simulink model "sim_battery_pack_simulink_18_11"  (R2021a)
settings: Solver=FixedStepAuto  StartTime=0.0  StopTime=3460.480  FixedStep=0.01  RelTol=1e-3
values from neighbouring files (symbols this model uses):
  Af = 1.4*1.6    (= 2.24)    [battery_pack_init_18_11.m]
  b = 0.002    [battery_pack_init_18_11.m]
  Batt_Eff = .98    (= 0.98)    [battery_pack_init_18_11.m]
  Batt_Ene_Cap = 7.37    [battery_pack_init_18_11.m]
  cd = 0.45    [battery_pack_init_18_11.m]
  dt = 0.01    [battery_pack_init_18_11.m]
  g = 9.81    [battery_pack_init_18_11.m]
  Gr = 5.75*.85    (= 4.8875)    [battery_pack_init_18_11.m]
  Grade = 7    [battery_pack_init_18_11.m]
  Ini_SOC = 100    [battery_pack_init_18_11.m]
  kappa = 0.1    [battery_pack_init_18_11.m]
  M = M_k+M_P    (= 445)    [battery_pack_init_18_11.m]
  M_Trq = T_m    [battery_pack_init_18_11.m]
  M_w = w_m    [battery_pack_init_18_11.m]
  Mot_Eff = .9    (= 0.9)    [battery_pack_init_18_11.m]
  mu = 0.016    [battery_pack_init_18_11.m]
  Np = 7    [battery_pack_init_18_11.m]
  Ns = 12    [battery_pack_init_18_11.m]
  Qgain = 1    [battery_pack_init_18_11.m]
  R0 = zeros(numpoles,1)    [battery_pack_init_18_11.m]
  R0Param = getParamESC('R0Param',T,cell_model)    [battery_pack_init_18_11.m]
  R_w = .3048/2    (= 0.1524)    [battery_pack_init_18_11.m]
  Re_spe_max = 50*5/18    (= 13.8888888889)    [battery_pack_init_18_11.m]
  Re_spe_min = 0*5/18    (= 0)    [battery_pack_init_18_11.m]
  rho = 1.225    [battery_pack_init_18_11.m]
  rt = .0008    (= 0.0008)    [battery_pack_init_18_11.m]
  T = 40    [battery_pack_init_18_11.m]
  T_MIDC = T_MIDC(1:72)    [battery_pack_init_18_11.m]
  Trans_Eff = .95    (= 0.95)    [battery_pack_init_18_11.m]
  V_MIDC = V_MIDC(1:72)    [battery_pack_init_18_11.m]
  Z0 = 0.75 + (1-0.75).*rand(1,Np)    [battery_pack_init_18_11.m]
undefined symbols (not defined in the file or in its folder): cell_model, FLbattery, gain, iload, sigbuilder_block, VMIDC
libraries: simulink x16, autolibshared x2, pid_lib x1, simulink_extras x1
(part 2 of 17)

== system sim_battery_pack_simulink_18_11/SCM3/cell2 ==
  ik1 : Inport
  Constant : Constant  Value=R0
  Constant1 : Constant  Value=dt
  Constant2 : Constant  Value=T
  States : Scope  NumInputPorts=2
  Unit Delay : UnitDelay  InitialCondition=Z0(2,3)  SampleTime=-1  HasFrameUpgradeWarning=on
  Unit Delay1 : UnitDelay  SampleTime=-1  HasFrameUpgradeWarning=on
  Voltage : Scope  NumInputPorts=2
  cell_model : MATLAB Function  TreatAsAtomicUnit=on
  V1 : Outport
  Z1 : Outport  Port=2
  irc1 : Outport  Port=3
  wires:
  cell_model/4(OCV) -> Voltage/2
  ik1/1 -> cell_model/6(ik)
  cell_model/3(zkc) -> Z1/1, Unit Delay/1, States/1
  cell_model/1(vk) -> V1/1, Voltage/1
  Constant1/1 -> cell_model/2(deltaT)
  Constant2/1 -> cell_model/1(T)
  Unit Delay/1 -> cell_model/4(zkp)
  cell_model/2(irkc) -> irc1/1, Unit Delay1/1, States/2
  Unit Delay1/1 -> cell_model/5(irkp)
  Constant/1 -> cell_model/3(iR0)

== system sim_battery_pack_simulink_18_11/SCM3/cell3 ==
  ik1 : Inport
  Constant : Constant  Value=R0
  Constant1 : Constant  Value=dt
  Constant2 : Constant  Value=T
  States : Scope  NumInputPorts=2
  Unit Delay : UnitDelay  InitialCondition=Z0(3,3)  SampleTime=-1  HasFrameUpgradeWarning=on
  Unit Delay1 : UnitDelay  SampleTime=-1  HasFrameUpgradeWarning=on
  Voltage : Scope  NumInputPorts=2
  cell_model : MATLAB Function  TreatAsAtomicUnit=on
  V1 : Outport
  Z1 : Outport  Port=2
  irc1 : Outport  Port=3
  wires:
  Constant/1 -> cell_model/3(iR0)
  Unit Delay1/1 -> cell_model/5(irkp)
  cell_model/2(irkc) -> States/2, Unit Delay1/1, irc1/1
  Unit Delay/1 -> cell_model/4(zkp)
  Constant2/1 -> cell_model/1(T)
  Constant1/1 -> cell_model/2(deltaT)
  cell_model/1(vk) -> Voltage/1, V1/1
  cell_model/3(zkc) -> States/1, Unit Delay/1, Z1/1
  ik1/1 -> cell_model/6(ik)
  cell_model/4(OCV) -> Voltage/2

== system sim_battery_pack_simulink_18_11/SCM3/cell4 ==
  ik1 : Inport
  Constant : Constant  Value=R0
  Constant1 : Constant  Value=dt
  Constant2 : Constant  Value=T
  States : Scope  NumInputPorts=2
  Unit Delay : UnitDelay  InitialCondition=Z0(4,3)  SampleTime=-1  HasFrameUpgradeWarning=on
  Unit Delay1 : UnitDelay  SampleTime=-1  HasFrameUpgradeWarning=on
  Voltage : Scope  NumInputPorts=2
  cell_model : MATLAB Function  TreatAsAtomicUnit=on
  V1 : Outport
  Z1 : Outport  Port=2
  irc1 : Outport  Port=3
  wires:
  Constant/1 -> cell_model/3(iR0)
  Unit Delay1/1 -> cell_model/5(irkp)
  cell_model/2(irkc) -> States/2, Unit Delay1/1, irc1/1
  Unit Delay/1 -> cell_model/4(zkp)
  Constant2/1 -> cell_model/1(T)
  Constant1/1 -> cell_model/2(deltaT)
  cell_model/1(vk) -> Voltage/1, V1/1
  cell_model/3(zkc) -> States/1, Unit Delay/1, Z1/1
  ik1/1 -> cell_model/6(ik)
  cell_model/4(OCV) -> Voltage/2

== system sim_battery_pack_simulink_18_11/SCM3/cell5 ==
  ik1 : Inport
  Constant : Constant  Value=R0
  Constant1 : Constant  Value=dt
  Constant2 : Constant  Value=T
  States : Scope  NumInputPorts=2
  Unit Delay : UnitDelay  InitialCondition=Z0(5,3)  SampleTime=-1  HasFrameUpgradeWarning=on
  Unit Delay1 : UnitDelay  SampleTime=-1  HasFrameUpgradeWarning=on
  Voltage : Scope  NumInputPorts=2
  cell_model : MATLAB Function  TreatAsAtomicUnit=on
  V1 : Outport
  Z1 : Outport  Port=2
  irc1 : Outport  Port=3
  wires:
  cell_model/4(OCV) -> Voltage/2
  ik1/1 -> cell_model/6(ik)
  cell_model/3(zkc) -> Z1/1, Unit Delay/1, States/1
  cell_model/1(vk) -> V1/1, Voltage/1
  Constant1/1 -> cell_model/2(deltaT)
  Constant2/1 -> cell_model/1(T)
  Unit Delay/1 -> cell_model/4(zkp)
  cell_model/2(irkc) -> irc1/1, Unit Delay1/1, States/2
  Unit Delay1/1 -> cell_model/5(irkp)
  Constant/1 -> cell_model/3(iR0)

== system sim_battery_pack_simulink_18_11/SCM3/cell6 ==
  ik1 : Inport
  Constant : Constant  Value=R0
  Constant1 : Constant  Value=dt
  Constant2 : Constant  Value=T
  States : Scope  NumInputPorts=2
  Unit Delay : UnitDelay  InitialCondition=Z0(6,3)  SampleTime=-1  HasFrameUpgradeWarning=on
  Unit Delay1 : UnitDelay  SampleTime=-1  HasFrameUpgradeWarning=on
  Voltage : Scope  NumInputPorts=2
  cell_model : MATLAB Function  TreatAsAtomicUnit=on
  V1 : Outport
  Z1 : Outport  Port=2
  irc1 : Outport  Port=3
  wires:
  cell_model/4(OCV) -> Voltage/2
  ik1/1 -> cell_model/6(ik)
  cell_model/3(zkc) -> Z1/1, Unit Delay/1, States/1
  cell_model/1(vk) -> V1/1, Voltage/1
  Constant1/1 -> cell_model/2(deltaT)
  Constant2/1 -> cell_model/1(T)
  Unit Delay/1 -> cell_model/4(zkp)
  cell_model/2(irkc) -> irc1/1, Unit Delay1/1, States/2
  Unit Delay1/1 -> cell_model/5(irkp)
  Constant/1 -> cell_model/3(iR0)

== system sim_battery_pack_simulink_18_11/SCM3/cell7 ==
  ik1 : Inport
  Constant : Constant  Value=R0
  Constant1 : Constant  Value=dt
  Constant2 : Constant  Value=T
  States : Scope  NumInputPorts=2
  Unit Delay : UnitDelay  InitialCondition=Z0(7,3)  SampleTime=-1  HasFrameUpgradeWarning=on
  Unit Delay1 : UnitDelay  SampleTime=-1  HasFrameUpgradeWarning=on
  Voltage : Scope  NumInputPorts=2
  cell_model : MATLAB Function  TreatAsAtomicUnit=on
  V1 : Outport
  Z1 : Outport  Port=2
  irc1 : Outport  Port=3
  wires:
  Constant/1 -> cell_model/3(iR0)
  Unit Delay1/1 -> cell_model/5(irkp)
  cell_model/2(irkc) -> States/2, Unit Delay1/1, irc1/1
  Unit Delay/1 -> cell_model/4(zkp)
  Constant2/1 -> cell_model/1(T)
  Constant1/1 -> cell_model/2(deltaT)
  cell_model/1(vk) -> Voltage/1, V1/1
  cell_model/3(zkc) -> States/1, Unit Delay/1, Z1/1
  ik1/1 -> cell_model/6(ik)
  cell_model/4(OCV) -> Voltage/2

== system sim_battery_pack_simulink_18_11/SCM3/cell8 ==
  ik1 : Inport
  Constant : Constant  Value=R0
  Constant1 : Constant  Value=dt
  Constant2 : Constant  Value=T
  States : Scope  NumInputPorts=2
  Unit Delay : UnitDelay  InitialCondition=Z0(8,3)  SampleTime=-1  HasFrameUpgradeWarning=on
  Unit Delay1 : UnitDelay  SampleTime=-1  HasFrameUpgradeWarning=on
  Voltage : Scope  NumInputPorts=2
  cell_model : MATLAB Function  TreatAsAtomicUnit=on
  V1 : Outport
  Z1 : Outport  Port=2
  irc1 : Outport  Port=3
  wires:
  cell_model/4(OCV) -> Voltage/2
  ik1/1 -> cell_model/6(ik)
  cell_model/3(zkc) -> Z1/1, Unit Delay/1, States/1
  cell_model/1(vk) -> V1/1, Voltage/1
  Constant1/1 -> cell_model/2(deltaT)
  Constant2/1 -> cell_model/1(T)
  Unit Delay/1 -> cell_model/4(zkp)
  cell_model/2(irkc) -> irc1/1, Unit Delay1/1, States/2
  Unit Delay1/1 -> cell_model/5(irkp)
  Constant/1 -> cell_model/3(iR0)

== system sim_battery_pack_simulink_18_11/SCM3/cell9 ==
  ik1 : Inport
  Constant : Constant  Value=R0
  Constant1 : Constant  Value=dt
  Constant2 : Constant  Value=T
  States : Scope  NumInputPorts=2
  Unit Delay : UnitDelay  InitialCondition=Z0(9,3)  SampleTime=-1  HasFrameUpgradeWarning=on
  Unit Delay1 : UnitDelay  SampleTime=-1  HasFrameUpgradeWarning=on
  Voltage : Scope  NumInputPorts=2
  cell_model : MATLAB Function  TreatAsAtomicUnit=on
  V1 : Outport
  Z1 : Outport  Port=2
  irc1 : Outport  Port=3
  wires:
  Constant/1 -> cell_model/3(iR0)
  Unit Delay1/1 -> cell_model/5(irkp)
  cell_model/2(irkc) -> States/2, Unit Delay1/1, irc1/1
  Unit Delay/1 -> cell_model/4(zkp)
  Constant2/1 -> cell_model/1(T)
  Constant1/1 -> cell_model/2(deltaT)
  cell_model/1(vk) -> Voltage/1, V1/1
  cell_model/3(zkc) -> States/1, Unit Delay/1, Z1/1
  ik1/1 -> cell_model/6(ik)
  cell_model/4(OCV) -> Voltage/2

== system sim_battery_pack_simulink_18_11/SCM4/cell1 ==
  ik1 : Inport
  Constant : Constant  Value=R0
  Constant1 : Constant  Value=dt
  Constant2 : Constant  Value=T
  States : Scope  NumInputPorts=2
  Unit Delay : UnitDelay  InitialCondition=Z0(1,4)  SampleTime=-1  HasFrameUpgradeWarning=on
  Unit Delay1 : UnitDelay  SampleTime=-1  HasFrameUpgradeWarning=on
  Voltage : Scope  NumInputPorts=2
  cell_model : MATLAB Function  TreatAsAtomicUnit=on
  V1 : Outport
  Z1 : Outport  Port=2
  irc1 : Outport  Port=3
  wires:
  Constant/1 -> cell_model/3(iR0)
  Unit Delay1/1 -> cell_model/5(irkp)
  cell_model/2(irkc) -> States/2, Unit Delay1/1, irc1/1
  Unit Delay/1 -> cell_model/4(zkp)
  Constant2/1 -> cell_model/1(T)
  Constant1/1 -> cell_model/2(deltaT)
  cell_model/1(vk) -> Voltage/1, V1/1
  cell_model/3(zkc) -> States/1, Unit Delay/1, Z1/1
  ik1/1 -> cell_model/6(ik)
  cell_model/4(OCV) -> Voltage/2

== system sim_battery_pack_simulink_18_11/SCM4/cell10 ==
  ik1 : Inport
  Constant : Constant  Value=R0
  Constant1 : Constant  Value=dt
  Constant2 : Constant  Value=T
  States : Scope  NumInputPorts=2
  Unit Delay : UnitDelay  InitialCondition=Z0(10,4)  SampleTime=-1  HasFrameUpgradeWarning=on
  Unit Delay1 : UnitDelay  SampleTime=-1  HasFrameUpgradeWarning=on
  Voltage : Scope  NumInputPorts=2
  cell_model : MATLAB Function  TreatAsAtomicUnit=on
  V1 : Outport
  Z1 : Outport  Port=2
  irc1 : Outport  Port=3
  wires:
  Constant/1 -> cell_model/3(iR0)
  Unit Delay1/1 -> cell_model/5(irkp)
  cell_model/2(irkc) -> States/2, Unit Delay1/1, irc1/1
  Unit Delay/1 -> cell_model/4(zkp)
  Constant2/1 -> cell_model/1(T)
  Constant1/1 -> cell_model/2(deltaT)
  cell_model/1(vk) -> Voltage/1, V1/1
  cell_model/3(zkc) -> States/1, Unit Delay/1, Z1/1
  ik1/1 -> cell_model/6(ik)
  cell_model/4(OCV) -> Voltage/2

== system sim_battery_pack_simulink_18_11/SCM4/cell11 ==
  ik1 : Inport
  Constant : Constant  Value=R0
  Constant1 : Constant  Value=dt
  Constant2 : Constant  Value=T
  States : Scope  NumInputPorts=2
  Unit Delay : UnitDelay  InitialCondition=Z0(11,4)  SampleTime=-1  HasFrameUpgradeWarning=on
  Unit Delay1 : UnitDelay  SampleTime=-1  HasFrameUpgradeWarning=on
  Voltage : Scope  NumInputPorts=2
  cell_model : MATLAB Function  TreatAsAtomicUnit=on
  V1 : Outport
  Z1 : Outport  Port=2
  irc1 : Outport  Port=3
  wires:
  cell_model/4(OCV) -> Voltage/2
  ik1/1 -> cell_model/6(ik)
  cell_model/3(zkc) -> Z1/1, Unit Delay/1, States/1
  cell_model/1(vk) -> V1/1, Voltage/1
  Constant1/1 -> cell_model/2(deltaT)
  Constant2/1 -> cell_model/1(T)
  Unit Delay/1 -> cell_model/4(zkp)
  cell_model/2(irkc) -> irc1/1, Unit Delay1/1, States/2
  Unit Delay1/1 -> cell_model/5(irkp)
  Constant/1 -> cell_model/3(iR0)

== system sim_battery_pack_simulink_18_11/SCM4/cell12 ==
  ik1 : Inport
  Constant : Constant  Value=R0
  Constant1 : Constant  Value=dt
  Constant2 : Constant  Value=T
  States : Scope  NumInputPorts=2
  Unit Delay : UnitDelay  InitialCondition=Z0(12,4)  SampleTime=-1  HasFrameUpgradeWarning=on
  Unit Delay1 : UnitDelay  SampleTime=-1  HasFrameUpgradeWarning=on
  Voltage : Scope  NumInputPorts=2
  cell_model : MATLAB Function  TreatAsAtomicUnit=on
  V1 : Outport
  Z1 : Outport  Port=2
  irc1 : Outport  Port=3
  wires:
  cell_model/4(OCV) -> Voltage/2
  ik1/1 -> cell_model/6(ik)
  cell_model/3(zkc) -> Z1/1, Unit Delay/1, States/1
  cell_model/1(vk) -> V1/1, Voltage/1
  Constant1/1 -> cell_model/2(deltaT)
  Constant2/1 -> cell_model/1(T)
  Unit Delay/1 -> cell_model/4(zkp)
  cell_model/2(irkc) -> irc1/1, Unit Delay1/1, States/2
  Unit Delay1/1 -> cell_model/5(irkp)
  Constant/1 -> cell_model/3(iR0)

== system sim_battery_pack_simulink_18_11/SCM4/cell2 ==
  ik1 : Inport
  Constant : Constant  Value=R0
  Constant1 : Constant  Value=dt
  Constant2 : Constant  Value=T
  States : Scope  NumInputPorts=2
  Unit Delay : UnitDelay  InitialCondition=Z0(2,4)  SampleTime=-1  HasFrameUpgradeWarning=on
  Unit Delay1 : UnitDelay  SampleTime=-1  HasFrameUpgradeWarning=on
  Voltage : Scope  NumInputPorts=2
  cell_model : MATLAB Function  TreatAsAtomicUnit=on
  V1 : Outport
  Z1 : Outport  Port=2
  irc1 : Outport  Port=3
  wires:
  Constant/1 -> cell_model/3(iR0)
  Unit Delay1/1 -> cell_model/5(irkp)
  cell_model/2(irkc) -> States/2, Unit Delay1/1, irc1/1
  Unit Delay/1 -> cell_model/4(zkp)
  Constant2/1 -> cell_model/1(T)
  Constant1/1 -> cell_model/2(deltaT)
  cell_model/1(vk) -> Voltage/1, V1/1
  cell_model/3(zkc) -> States/1, Unit Delay/1, Z1/1
  ik1/1 -> cell_model/6(ik)
  cell_model/4(OCV) -> Voltage/2

== system sim_battery_pack_simulink_18_11/SCM4/cell3 ==
  ik1 : Inport
  Constant : Constant  Value=R0
  Constant1 : Constant  Value=dt
  Constant2 : Constant  Value=T
  States : Scope  NumInputPorts=2
  Unit Delay : UnitDelay  InitialCondition=Z0(3,4)  SampleTime=-1  HasFrameUpgradeWarning=on
  Unit Delay1 : UnitDelay  SampleTime=-1  HasFrameUpgradeWarning=on
  Voltage : Scope  NumInputPorts=2
  cell_model : MATLAB Function  TreatAsAtomicUnit=on
  V1 : Outport
  Z1 : Outport  Port=2
  irc1 : Outport  Port=3
  wires:
  cell_model/4(OCV) -> Voltage/2
  ik1/1 -> cell_model/6(ik)
  cell_model/3(zkc) -> Z1/1, Unit Delay/1, States/1
  cell_model/1(vk) -> V1/1, Voltage/1
  Constant1/1 -> cell_model/2(deltaT)
  Constant2/1 -> cell_model/1(T)
  Unit Delay/1 -> cell_model/4(zkp)
  cell_model/2(irkc) -> irc1/1, Unit Delay1/1, States/2
  Unit Delay1/1 -> cell_model/5(irkp)
  Constant/1 -> cell_model/3(iR0)

== system sim_battery_pack_simulink_18_11/SCM4/cell4 ==
  ik1 : Inport
  Constant : Constant  Value=R0
  Constant1 : Constant  Value=dt
  Constant2 : Constant  Value=T
  States : Scope  NumInputPorts=2
  Unit Delay : UnitDelay  InitialCondition=Z0(4,4)  SampleTime=-1  HasFrameUpgradeWarning=on
  Unit Delay1 : UnitDelay  SampleTime=-1  HasFrameUpgradeWarning=on
  Voltage : Scope  NumInputPorts=2
  cell_model : MATLAB Function  TreatAsAtomicUnit=on
  V1 : Outport
  Z1 : Outport  Port=2
  irc1 : Outport  Port=3
  wires:
  cell_model/4(OCV) -> Voltage/2
  ik1/1 -> cell_model/6(ik)
  cell_model/3(zkc) -> Z1/1, Unit Delay/1, States/1
  cell_model/1(vk) -> V1/1, Voltage/1
  Constant1/1 -> cell_model/2(deltaT)
  Constant2/1 -> cell_model/1(T)
  Unit Delay/1 -> cell_model/4(zkp)
  cell_model/2(irkc) -> irc1/1, Unit Delay1/1, States/2
  Unit Delay1/1 -> cell_model/5(irkp)
  Constant/1 -> cell_model/3(iR0)

== system sim_battery_pack_simulink_18_11/SCM4/cell5 ==
  ik1 : Inport
  Constant : Constant  Value=R0
  Constant1 : Constant  Value=dt
  Constant2 : Constant  Value=T
  States : Scope  NumInputPorts=2
  Unit Delay : UnitDelay  InitialCondition=Z0(5,4)  SampleTime=-1  HasFrameUpgradeWarning=on
  Unit Delay1 : UnitDelay  SampleTime=-1  HasFrameUpgradeWarning=on
  Voltage : Scope  NumInputPorts=2
  cell_model : MATLAB Function  TreatAsAtomicUnit=on
  V1 : Outport
  Z1 : Outport  Port=2
  irc1 : Outport  Port=3
  wires:
  Constant/1 -> cell_model/3(iR0)
  Unit Delay1/1 -> cell_model/5(irkp)
  cell_model/2(irkc) -> States/2, Unit Delay1/1, irc1/1
  Unit Delay/1 -> cell_model/4(zkp)
  Constant2/1 -> cell_model/1(T)
  Constant1/1 -> cell_model/2(deltaT)
  cell_model/1(vk) -> Voltage/1, V1/1
  cell_model/3(zkc) -> States/1, Unit Delay/1, Z1/1
  ik1/1 -> cell_model/6(ik)
  cell_model/4(OCV) -> Voltage/2

== system sim_battery_pack_simulink_18_11/SCM4/cell6 ==
  ik1 : Inport
  Constant : Constant  Value=R0
  Constant1 : Constant  Value=dt
  Constant2 : Constant  Value=T
  States : Scope  NumInputPorts=2
  Unit Delay : UnitDelay  InitialCondition=Z0(6,4)  SampleTime=-1  HasFrameUpgradeWarning=on
  Unit Delay1 : UnitDelay  SampleTime=-1  HasFrameUpgradeWarning=on
  Voltage : Scope  NumInputPorts=2
  cell_model : MATLAB Function  TreatAsAtomicUnit=on
  V1 : Outport
  Z1 : Outport  Port=2
  irc1 : Outport  Port=3
  wires:
  Constant/1 -> cell_model/3(iR0)
  Unit Delay1/1 -> cell_model/5(irkp)
  cell_model/2(irkc) -> States/2, Unit Delay1/1, irc1/1
  Unit Delay/1 -> cell_model/4(zkp)
  Constant2/1 -> cell_model/1(T)
  Constant1/1 -> cell_model/2(deltaT)
  cell_model/1(vk) -> Voltage/1, V1/1
  cell_model/3(zkc) -> States/1, Unit Delay/1, Z1/1
  ik1/1 -> cell_model/6(ik)
  cell_model/4(OCV) -> Voltage/2

== system sim_battery_pack_simulink_18_11/SCM4/cell7 ==
  ik1 : Inport
  Constant : Constant  Value=R0
  Constant1 : Constant  Value=dt
  Constant2 : Constant  Value=T
  States : Scope  NumInputPorts=2
  Unit Delay : UnitDelay  InitialCondition=Z0(7,4)  SampleTime=-1  HasFrameUpgradeWarning=on
  Unit Delay1 : UnitDelay  SampleTime=-1  HasFrameUpgradeWarning=on
  Voltage : Scope  NumInputPorts=2
  cell_model : MATLAB Function  TreatAsAtomicUnit=on
  V1 : Outport
  Z1 : Outport  Port=2
  irc1 : Outport  Port=3
  wires:
  cell_model/4(OCV) -> Voltage/2
  ik1/1 -> cell_model/6(ik)
  cell_model/3(zkc) -> Z1/1, Unit Delay/1, States/1
  cell_model/1(vk) -> V1/1, Voltage/1
  Constant1/1 -> cell_model/2(deltaT)
  Constant2/1 -> cell_model/1(T)
  Unit Delay/1 -> cell_model/4(zkp)
  cell_model/2(irkc) -> irc1/1, Unit Delay1/1, States/2
  Unit Delay1/1 -> cell_model/5(irkp)
  Constant/1 -> cell_model/3(iR0)

== system sim_battery_pack_simulink_18_11/SCM4/cell8 ==
  ik1 : Inport
  Constant : Constant  Value=R0
  Constant1 : Constant  Value=dt
  Constant2 : Constant  Value=T
  States : Scope  NumInputPorts=2
  Unit Delay : UnitDelay  InitialCondition=Z0(8,4)  SampleTime=-1  HasFrameUpgradeWarning=on
  Unit Delay1 : UnitDelay  SampleTime=-1  HasFrameUpgradeWarning=on
  Voltage : Scope  NumInputPorts=2
  cell_model : MATLAB Function  TreatAsAtomicUnit=on
  V1 : Outport
  Z1 : Outport  Port=2
  irc1 : Outport  Port=3
  wires:
  Constant/1 -> cell_model/3(iR0)
  Unit Delay1/1 -> cell_model/5(irkp)
  cell_model/2(irkc) -> States/2, Unit Delay1/1, irc1/1
  Unit Delay/1 -> cell_model/4(zkp)
  Constant2/1 -> cell_model/1(T)
  Constant1/1 -> cell_model/2(deltaT)
  cell_model/1(vk) -> Voltage/1, V1/1
  cell_model/3(zkc) -> States/1, Unit Delay/1, Z1/1
  ik1/1 -> cell_model/6(ik)
  cell_model/4(OCV) -> Voltage/2

== system sim_battery_pack_simulink_18_11/SCM4/cell9 ==
  ik1 : Inport
  Constant : Constant  Value=R0
  Constant1 : Constant  Value=dt
  Constant2 : Constant  Value=T
  States : Scope  NumInputPorts=2
  Unit Delay : UnitDelay  InitialCondition=Z0(9,4)  SampleTime=-1  HasFrameUpgradeWarning=on
  Unit Delay1 : UnitDelay  SampleTime=-1  HasFrameUpgradeWarning=on
  Voltage : Scope  NumInputPorts=2
  cell_model : MATLAB Function  TreatAsAtomicUnit=on
  V1 : Outport
  Z1 : Outport  Port=2
  irc1 : Outport  Port=3
  wires:
  cell_model/4(OCV) -> Voltage/2
  ik1/1 -> cell_model/6(ik)
  cell_model/3(zkc) -> Z1/1, Unit Delay/1, States/1
  cell_model/1(vk) -> V1/1, Voltage/1
  Constant1/1 -> cell_model/2(deltaT)
  Constant2/1 -> cell_model/1(T)
  Unit Delay/1 -> cell_model/4(zkp)
  cell_model/2(irkc) -> irc1/1, Unit Delay1/1, States/2
  Unit Delay1/1 -> cell_model/5(irkp)
  Constant/1 -> cell_model/3(iR0)

== system sim_battery_pack_simulink_18_11/SCM5/cell1 ==
  ik1 : Inport
  Constant : Constant  Value=R0
  Constant1 : Constant  Value=dt
  Constant2 : Constant  Value=T
  States : Scope  NumInputPorts=2
  Unit Delay : UnitDelay  InitialCondition=Z0(1,5)  SampleTime=-1  HasFrameUpgradeWarning=on
  Unit Delay1 : UnitDelay  SampleTime=-1  HasFrameUpgradeWarning=on
  Voltage : Scope  NumInputPorts=2
  cell_model : MATLAB Function  TreatAsAtomicUnit=on
  V1 : Outport
  Z1 : Outport  Port=2
  irc1 : Outport  Port=3
  wires:
  Constant/1 -> cell_model/3(iR0)
  Unit Delay1/1 -> cell_model/5(irkp)
  cell_model/2(irkc) -> States/2, Unit Delay1/1, irc1/1
  Unit Delay/1 -> cell_model/4(zkp)
  Constant2/1 -> cell_model/1(T)
  Constant1/1 -> cell_model/2(deltaT)
  cell_model/1(vk) -> Voltage/1, V1/1
  cell_model/3(zkc) -> States/1, Unit Delay/1, Z1/1
  ik1/1 -> cell_model/6(ik)
  cell_model/4(OCV) -> Voltage/2

== system sim_battery_pack_simulink_18_11/SCM5/cell10 ==
  ik1 : Inport
  Constant : Constant  Value=R0
  Constant1 : Constant  Value=dt
  Constant2 : Constant  Value=T
  States : Scope  NumInputPorts=2
  Unit Delay : UnitDelay  InitialCondition=Z0(10,5)  SampleTime=-1  HasFrameUpgradeWarning=on
  Unit Delay1 : UnitDelay  SampleTime=-1  HasFrameUpgradeWarning=on
  Voltage : Scope  NumInputPorts=2
  cell_model : MATLAB Function  TreatAsAtomicUnit=on
  V1 : Outport
  Z1 : Outport  Port=2
  irc1 : Outport  Port=3
  wires:
  Constant/1 -> cell_model/3(iR0)
  Unit Delay1/1 -> cell_model/5(irkp)
  cell_model/2(irkc) -> States/2, Unit Delay1/1, irc1/1
  Unit Delay/1 -> cell_model/4(zkp)
  Constant2/1 -> cell_model/1(T)
  Constant1/1 -> cell_model/2(deltaT)
  cell_model/1(vk) -> Voltage/1, V1/1
  cell_model/3(zkc) -> States/1, Unit Delay/1, Z1/1
  ik1/1 -> cell_model/6(ik)
  cell_model/4(OCV) -> Voltage/2

== system sim_battery_pack_simulink_18_11/SCM5/cell11 ==
  ik1 : Inport
  Constant : Constant  Value=R0
  Constant1 : Constant  Value=dt
  Constant2 : Constant  Value=T
  States : Scope  NumInputPorts=2
  Unit Delay : UnitDelay  InitialCondition=Z0(11,5)  SampleTime=-1  HasFrameUpgradeWarning=on
  Unit Delay1 : UnitDelay  SampleTime=-1  HasFrameUpgradeWarning=on
  Voltage : Scope  NumInputPorts=2
  cell_model : MATLAB Function  TreatAsAtomicUnit=on
  V1 : Outport
  Z1 : Outport  Port=2
  irc1 : Outport  Port=3
  wires:
  cell_model/4(OCV) -> Voltage/2
  ik1/1 -> cell_model/6(ik)
  cell_model/3(zkc) -> Z1/1, Unit Delay/1, States/1
  cell_model/1(vk) -> V1/1, Voltage/1
  Constant1/1 -> cell_model/2(deltaT)
  Constant2/1 -> cell_model/1(T)
  Unit Delay/1 -> cell_model/4(zkp)
  cell_model/2(irkc) -> irc1/1, Unit Delay1/1, States/2
  Unit Delay1/1 -> cell_model/5(irkp)
  Constant/1 -> cell_model/3(iR0)

== system sim_battery_pack_simulink_18_11/SCM5/cell12 ==
  ik1 : Inport
  Constant : Constant  Value=R0
  Constant1 : Constant  Value=dt
  Constant2 : Constant  Value=T
  States : Scope  NumInputPorts=2
  Unit Delay : UnitDelay  InitialCondition=Z0(12,5)  SampleTime=-1  HasFrameUpgradeWarning=on
  Unit Delay1 : UnitDelay  SampleTime=-1  HasFrameUpgradeWarning=on
  Voltage : Scope  NumInputPorts=2
  cell_model : MATLAB Function  TreatAsAtomicUnit=on
  V1 : Outport
  Z1 : Outport  Port=2
  irc1 : Outport  Port=3
  wires:
  cell_model/4(OCV) -> Voltage/2
  ik1/1 -> cell_model/6(ik)
  cell_model/3(zkc) -> Z1/1, Unit Delay/1, States/1
  cell_model/1(vk) -> V1/1, Voltage/1
  Constant1/1 -> cell_model/2(deltaT)
  Constant2/1 -> cell_model/1(T)
  Unit Delay/1 -> cell_model/4(zkp)
  cell_model/2(irkc) -> irc1/1, Unit Delay1/1, States/2
  Unit Delay1/1 -> cell_model/5(irkp)
  Constant/1 -> cell_model/3(iR0)

== system sim_battery_pack_simulink_18_11/SCM5/cell2 ==
  ik1 : Inport
  Constant : Constant  Value=R0
  Constant1 : Constant  Value=dt
  Constant2 : Constant  Value=T
  States : Scope  NumInputPorts=2
  Unit Delay : UnitDelay  InitialCondition=Z0(2,5)  SampleTime=-1  HasFrameUpgradeWarning=on
  Unit Delay1 : UnitDelay  SampleTime=-1  HasFrameUpgradeWarning=on
  Voltage : Scope  NumInputPorts=2
  cell_model : MATLAB Function  TreatAsAtomicUnit=on
  V1 : Outport
  Z1 : Outport  Port=2
  irc1 : Outport  Port=3
  wires:
  Constant/1 -> cell_model/3(iR0)
  Unit Delay1/1 -> cell_model/5(irkp)
  cell_model/2(irkc) -> States/2, Unit Delay1/1, irc1/1
  Unit Delay/1 -> cell_model/4(zkp)
  Constant2/1 -> cell_model/1(T)
  Constant1/1 -> cell_model/2(deltaT)
  cell_model/1(vk) -> Voltage/1, V1/1
  cell_model/3(zkc) -> States/1, Unit Delay/1, Z1/1
  ik1/1 -> cell_model/6(ik)
  cell_model/4(OCV) -> Voltage/2

== system sim_battery_pack_simulink_18_11/SCM5/cell3 ==
  ik1 : Inport
  Constant : Constant  Value=R0
  Constant1 : Constant  Value=dt
  Constant2 : Constant  Value=T
  States : Scope  NumInputPorts=2
  Unit Delay : UnitDelay  InitialCondition=Z0(3,5)  SampleTime=-1  HasFrameUpgradeWarning=on
  Unit Delay1 : UnitDelay  SampleTime=-1  HasFrameUpgradeWarning=on
  Voltage : Scope  NumInputPorts=2
  cell_model : MATLAB Function  TreatAsAtomicUnit=on
  V1 : Outport
  Z1 : Outport  Port=2
  irc1 : Outport  Port=3
  wires:
  cell_model/4(OCV) -> Voltage/2
  ik1/1 -> cell_model/6(ik)
  cell_model/3(zkc) -> Z1/1, Unit Delay/1, States/1
  cell_model/1(vk) -> V1/1, Voltage/1
  Constant1/1 -> cell_model/2(deltaT)
  Constant2/1 -> cell_model/1(T)
  Unit Delay/1 -> cell_model/4(zkp)
  cell_model/2(irkc) -> irc1/1, Unit Delay1/1, States/2
  Unit Delay1/1 -> cell_model/5(irkp)
  Constant/1 -> cell_model/3(iR0)

== system sim_battery_pack_simulink_18_11/SCM5/cell4 ==
  ik1 : Inport
  Constant : Constant  Value=R0
  Constant1 : Constant  Value=dt
  Constant2 : Constant  Value=T
  States : Scope  NumInputPorts=2
  Unit Delay : UnitDelay  InitialCondition=Z0(4,5)  SampleTime=-1  HasFrameUpgradeWarning=on
  Unit Delay1 : UnitDelay  SampleTime=-1  HasFrameUpgradeWarning=on
  Voltage : Scope  NumInputPorts=2
  cell_model : MATLAB Function  TreatAsAtomicUnit=on
  V1 : Outport
  Z1 : Outport  Port=2
  irc1 : Outport  Port=3
  wires:
  cell_model/4(OCV) -> Voltage/2
  ik1/1 -> cell_model/6(ik)
  cell_model/3(zkc) -> Z1/1, Unit Delay/1, States/1
  cell_model/1(vk) -> V1/1, Voltage/1
  Constant1/1 -> cell_model/2(deltaT)
  Constant2/1 -> cell_model/1(T)
  Unit Delay/1 -> cell_model/4(zkp)
  cell_model/2(irkc) -> irc1/1, Unit Delay1/1, States/2
  Unit Delay1/1 -> cell_model/5(irkp)
  Constant/1 -> cell_model/3(iR0)

== system sim_battery_pack_simulink_18_11/SCM5/cell5 ==
  ik1 : Inport
  Constant : Constant  Value=R0
  Constant1 : Constant  Value=dt
  Constant2 : Constant  Value=T
  States : Scope  NumInputPorts=2
  Unit Delay : UnitDelay  InitialCondition=Z0(5,5)  SampleTime=-1  HasFrameUpgradeWarning=on
  Unit Delay1 : UnitDelay  SampleTime=-1  HasFrameUpgradeWarning=on
  Voltage : Scope  NumInputPorts=2
  cell_model : MATLAB Function  TreatAsAtomicUnit=on
  V1 : Outport
  Z1 : Outport  Port=2
  irc1 : Outport  Port=3
  wires:
  Constant/1 -> cell_model/3(iR0)
  Unit Delay1/1 -> cell_model/5(irkp)
  cell_model/2(irkc) -> States/2, Unit Delay1/1, irc1/1
  Unit Delay/1 -> cell_model/4(zkp)
  Constant2/1 -> cell_model/1(T)
  Constant1/1 -> cell_model/2(deltaT)
  cell_model/1(vk) -> Voltage/1, V1/1
  cell_model/3(zkc) -> States/1, Unit Delay/1, Z1/1
  ik1/1 -> cell_model/6(ik)
  cell_model/4(OCV) -> Voltage/2

== system sim_battery_pack_simulink_18_11/SCM5/cell6 ==
  ik1 : Inport
  Constant : Constant  Value=R0
  Constant1 : Constant  Value=dt
  Constant2 : Constant  Value=T
  States : Scope  NumInputPorts=2
  Unit Delay : UnitDelay  InitialCondition=Z0(6,5)  SampleTime=-1  HasFrameUpgradeWarning=on
  Unit Delay1 : UnitDelay  SampleTime=-1  HasFrameUpgradeWarning=on
  Voltage : Scope  NumInputPorts=2
  cell_model : MATLAB Function  TreatAsAtomicUnit=on
  V1 : Outport
  Z1 : Outport  Port=2
  irc1 : Outport  Port=3
  wires:
  Constant/1 -> cell_model/3(iR0)
  Unit Delay1/1 -> cell_model/5(irkp)
  cell_model/2(irkc) -> States/2, Unit Delay1/1, irc1/1
  Unit Delay/1 -> cell_model/4(zkp)
  Constant2/1 -> cell_model/1(T)
  Constant1/1 -> cell_model/2(deltaT)
  cell_model/1(vk) -> Voltage/1, V1/1
  cell_model/3(zkc) -> States/1, Unit Delay/1, Z1/1
  ik1/1 -> cell_model/6(ik)
  cell_model/4(OCV) -> Voltage/2

== system sim_battery_pack_simulink_18_11/SCM5/cell7 ==
  ik1 : Inport
  Constant : Constant  Value=R0
  Constant1 : Constant  Value=dt
  Constant2 : Constant  Value=T
  States : Scope  NumInputPorts=2
  Unit Delay : UnitDelay  InitialCondition=Z0(7,5)  SampleTime=-1  HasFrameUpgradeWarning=on
  Unit Delay1 : UnitDelay  SampleTime=-1  HasFrameUpgradeWarning=on
  Voltage : Scope  NumInputPorts=2
  cell_model : MATLAB Function  TreatAsAtomicUnit=on
  V1 : Outport
  Z1 : Outport  Port=2
  irc1 : Outport  Port=3
  wires:
  cell_model/4(OCV) -> Voltage/2
  ik1/1 -> cell_model/6(ik)
  cell_model/3(zkc) -> Z1/1, Unit Delay/1, States/1
  cell_model/1(vk) -> V1/1, Voltage/1
  Constant1/1 -> cell_model/2(deltaT)
  Constant2/1 -> cell_model/1(T)
  Unit Delay/1 -> cell_model/4(zkp)
  cell_model/2(irkc) -> irc1/1, Unit Delay1/1, States/2
  Unit Delay1/1 -> cell_model/5(irkp)
  Constant/1 -> cell_model/3(iR0)

== system sim_battery_pack_simulink_18_11/SCM5/cell8 ==
  ik1 : Inport
  Constant : Constant  Value=R0
  Constant1 : Constant  Value=dt
  Constant2 : Constant  Value=T
  States : Scope  NumInputPorts=2
  Unit Delay : UnitDelay  InitialCondition=Z0(8,5)  SampleTime=-1  HasFrameUpgradeWarning=on
  Unit Delay1 : UnitDelay  SampleTime=-1  HasFrameUpgradeWarning=on
  Voltage : Scope  NumInputPorts=2
  cell_model : MATLAB Function  TreatAsAtomicUnit=on
  V1 : Outport
  Z1 : Outport  Port=2
  irc1 : Outport  Port=3
  wires:
  Constant/1 -> cell_model/3(iR0)
  Unit Delay1/1 -> cell_model/5(irkp)
  cell_model/2(irkc) -> States/2, Unit Delay1/1, irc1/1
  Unit Delay/1 -> cell_model/4(zkp)
  Constant2/1 -> cell_model/1(T)
  Constant1/1 -> cell_model/2(deltaT)
  cell_model/1(vk) -> Voltage/1, V1/1
  cell_model/3(zkc) -> States/1, Unit Delay/1, Z1/1
  ik1/1 -> cell_model/6(ik)
  cell_model/4(OCV) -> Voltage/2

== system sim_battery_pack_simulink_18_11/SCM5/cell9 ==
  ik1 : Inport
  Constant : Constant  Value=R0
  Constant1 : Constant  Value=dt
  Constant2 : Constant  Value=T
  States : Scope  NumInputPorts=2
  Unit Delay : UnitDelay  InitialCondition=Z0(9,5)  SampleTime=-1  HasFrameUpgradeWarning=on
  Unit Delay1 : UnitDelay  SampleTime=-1  HasFrameUpgradeWarning=on
  Voltage : Scope  NumInputPorts=2
  cell_model : MATLAB Function  TreatAsAtomicUnit=on
  V1 : Outport
  Z1 : Outport  Port=2
  irc1 : Outport  Port=3
  wires:
  cell_model/4(OCV) -> Voltage/2
  ik1/1 -> cell_model/6(ik)
  cell_model/3(zkc) -> Z1/1, Unit Delay/1, States/1
  cell_model/1(vk) -> V1/1, Voltage/1
  Constant1/1 -> cell_model/2(deltaT)
  Constant2/1 -> cell_model/1(T)
  Unit Delay/1 -> cell_model/4(zkp)
  cell_model/2(irkc) -> irc1/1, Unit Delay1/1, States/2
  Unit Delay1/1 -> cell_model/5(irkp)
  Constant/1 -> cell_model/3(iR0)

== system sim_battery_pack_simulink_18_11/SCM6/cell1 ==
  ik1 : Inport
  Constant : Constant  Value=R0
  Constant1 : Constant  Value=dt
  Constant2 : Constant  Value=T
  States : Scope  NumInputPorts=2
  Unit Delay : UnitDelay  InitialCondition=Z0(1,6)  SampleTime=-1  HasFrameUpgradeWarning=on
  Unit Delay1 : UnitDelay  SampleTime=-1  HasFrameUpgradeWarning=on
  Voltage : Scope  NumInputPorts=2
  cell_model : MATLAB Function  TreatAsAtomicUnit=on
  V1 : Outport
  Z1 : Outport  Port=2
  irc1 : Outport  Port=3
  wires:
  Constant/1 -> cell_model/3(iR0)
  Unit Delay1/1 -> cell_model/5(irkp)
  cell_model/2(irkc) -> States/2, Unit Delay1/1, irc1/1
  Unit Delay/1 -> cell_model/4(zkp)
  Constant2/1 -> cell_model/1(T)
  Constant1/1 -> cell_model/2(deltaT)
  cell_model/1(vk) -> Voltage/1, V1/1
  cell_model/3(zkc) -> States/1, Unit Delay/1, Z1/1
  ik1/1 -> cell_model/6(ik)
  cell_model/4(OCV) -> Voltage/2

== system sim_battery_pack_simulink_18_11/SCM6/cell10 ==
  ik1 : Inport
  Constant : Constant  Value=R0
  Constant1 : Constant  Value=dt
  Constant2 : Constant  Value=T
  States : Scope  NumInputPorts=2
  Unit Delay : UnitDelay  InitialCondition=Z0(10,6)  SampleTime=-1  HasFrameUpgradeWarning=on
  Unit Delay1 : UnitDelay  SampleTime=-1  HasFrameUpgradeWarning=on
  Voltage : Scope  NumInputPorts=2
  cell_model : MATLAB Function  TreatAsAtomicUnit=on
  V1 : Outport
  Z1 : Outport  Port=2
  irc1 : Outport  Port=3
  wires:
  Constant/1 -> cell_model/3(iR0)
  Unit Delay1/1 -> cell_model/5(irkp)
  cell_model/2(irkc) -> States/2, Unit Delay1/1, irc1/1
  Unit Delay/1 -> cell_model/4(zkp)
  Constant2/1 -> cell_model/1(T)
  Constant1/1 -> cell_model/2(deltaT)
  cell_model/1(vk) -> Voltage/1, V1/1
  cell_model/3(zkc) -> States/1, Unit Delay/1, Z1/1
  ik1/1 -> cell_model/6(ik)
  cell_model/4(OCV) -> Voltage/2

== system sim_battery_pack_simulink_18_11/SCM6/cell11 ==
  ik1 : Inport
  Constant : Constant  Value=R0
  Constant1 : Constant  Value=dt
  Constant2 : Constant  Value=T
  States : Scope  NumInputPorts=2
  Unit Delay : UnitDelay  InitialCondition=Z0(11,6)  SampleTime=-1  HasFrameUpgradeWarning=on
  Unit Delay1 : UnitDelay  SampleTime=-1  HasFrameUpgradeWarning=on
  Voltage : Scope  NumInputPorts=2
  cell_model : MATLAB Function  TreatAsAtomicUnit=on
  V1 : Outport
  Z1 : Outport  Port=2
  irc1 : Outport  Port=3
  wires:
  cell_model/4(OCV) -> Voltage/2
  ik1/1 -> cell_model/6(ik)
  cell_model/3(zkc) -> Z1/1, Unit Delay/1, States/1
  cell_model/1(vk) -> V1/1, Voltage/1
  Constant1/1 -> cell_model/2(deltaT)
  Constant2/1 -> cell_model/1(T)
  Unit Delay/1 -> cell_model/4(zkp)
  cell_model/2(irkc) -> irc1/1, Unit Delay1/1, States/2
  Unit Delay1/1 -> cell_model/5(irkp)
  Constant/1 -> cell_model/3(iR0)

== system sim_battery_pack_simulink_18_11/SCM6/cell12 ==
  ik1 : Inport
  Constant : Constant  Value=R0
  Constant1 : Constant  Value=dt
  Constant2 : Constant  Value=T
  States : Scope  NumInputPorts=2
  Unit Delay : UnitDelay  InitialCondition=Z0(12,6)  SampleTime=-1  HasFrameUpgradeWarning=on
  Unit Delay1 : UnitDelay  SampleTime=-1  HasFrameUpgradeWarning=on
  Voltage : Scope  NumInputPorts=2
  cell_model : MATLAB Function  TreatAsAtomicUnit=on
  V1 : Outport
  Z1 : Outport  Port=2
  irc1 : Outport  Port=3
  wires:
  cell_model/4(OCV) -> Voltage/2
  ik1/1 -> cell_model/6(ik)
  cell_model/3(zkc) -> Z1/1, Unit Delay/1, States/1
  cell_model/1(vk) -> V1/1, Voltage/1
  Constant1/1 -> cell_model/2(deltaT)
  Constant2/1 -> cell_model/1(T)
  Unit Delay/1 -> cell_model/4(zkp)
  cell_model/2(irkc) -> irc1/1, Unit Delay1/1, States/2
  Unit Delay1/1 -> cell_model/5(irkp)
  Constant/1 -> cell_model/3(iR0)

== system sim_battery_pack_simulink_18_11/SCM6/cell2 ==
  ik1 : Inport
  Constant : Constant  Value=R0
  Constant1 : Constant  Value=dt
  Constant2 : Constant  Value=T
  States : Scope  NumInputPorts=2
  Unit Delay : UnitDelay  InitialCondition=Z0(2,6)  SampleTime=-1  HasFrameUpgradeWarning=on
  Unit Delay1 : UnitDelay  SampleTime=-1  HasFrameUpgradeWarning=on
  Voltage : Scope  NumInputPorts=2
  cell_model : MATLAB Function  TreatAsAtomicUnit=on
  V1 : Outport
  Z1 : Outport  Port=2
  irc1 : Outport  Port=3
  wires:
  Constant/1 -> cell_model/3(iR0)
  Unit Delay1/1 -> cell_model/5(irkp)
  cell_model/2(irkc) -> States/2, Unit Delay1/1, irc1/1
  Unit Delay/1 -> cell_model/4(zkp)
  Constant2/1 -> cell_model/1(T)
  Constant1/1 -> cell_model/2(deltaT)
  cell_model/1(vk) -> Voltage/1, V1/1
  cell_model/3(zkc) -> States/1, Unit Delay/1, Z1/1
  ik1/1 -> cell_model/6(ik)
  cell_model/4(OCV) -> Voltage/2

== system sim_battery_pack_simulink_18_11/SCM6/cell3 ==
  ik1 : Inport
  Constant : Constant  Value=R0
  Constant1 : Constant  Value=dt
  Constant2 : Constant  Value=T
  States : Scope  NumInputPorts=2
  Unit Delay : UnitDelay  InitialCondition=Z0(3,6)  SampleTime=-1  HasFrameUpgradeWarning=on
  Unit Delay1 : UnitDelay  SampleTime=-1  HasFrameUpgradeWarning=on
  Voltage : Scope  NumInputPorts=2
  cell_model : MATLAB Function  TreatAsAtomicUnit=on
  V1 : Outport
  Z1 : Outport  Port=2
  irc1 : Outport  Port=3
  wires:
  cell_model/4(OCV) -> Voltage/2
  ik1/1 -> cell_model/6(ik)
  cell_model/3(zkc) -> Z1/1, Unit Delay/1, States/1
  cell_model/1(vk) -> V1/1, Voltage/1
  Constant1/1 -> cell_model/2(deltaT)
  Constant2/1 -> cell_model/1(T)
  Unit Delay/1 -> cell_model/4(zkp)
  cell_model/2(irkc) -> irc1/1, Unit Delay1/1, States/2
  Unit Delay1/1 -> cell_model/5(irkp)
  Constant/1 -> cell_model/3(iR0)

== system sim_battery_pack_simulink_18_11/SCM6/cell4 ==
  ik1 : Inport
  Constant : Constant  Value=R0
  Constant1 : Constant  Value=dt
  Constant2 : Constant  Value=T
  States : Scope  NumInputPorts=2
  Unit Delay : UnitDelay  InitialCondition=Z0(4,6)  SampleTime=-1  HasFrameUpgradeWarning=on
  Unit Delay1 : UnitDelay  SampleTime=-1  HasFrameUpgradeWarning=on
  Voltage : Scope  NumInputPorts=2
  cell_model : MATLAB Function  TreatAsAtomicUnit=on
  V1 : Outport
  Z1 : Outport  Port=2
  irc1 : Outport  Port=3
  wires:
  cell_model/4(OCV) -> Voltage/2
  ik1/1 -> cell_model/6(ik)
  cell_model/3(zkc) -> Z1/1, Unit Delay/1, States/1
  cell_model/1(vk) -> V1/1, Voltage/1
  Constant1/1 -> cell_model/2(deltaT)
  Constant2/1 -> cell_model/1(T)
  Unit Delay/1 -> cell_model/4(zkp)
  cell_model/2(irkc) -> irc1/1, Unit Delay1/1, States/2
  Unit Delay1/1 -> cell_model/5(irkp)
  Constant/1 -> cell_model/3(iR0)

== system sim_battery_pack_simulink_18_11/SCM6/cell5 ==
  ik1 : Inport
  Constant : Constant  Value=R0
  Constant1 : Constant  Value=dt
  Constant2 : Constant  Value=T
  States : Scope  NumInputPorts=2
  Unit Delay : UnitDelay  InitialCondition=Z0(5,6)  SampleTime=-1  HasFrameUpgradeWarning=on
  Unit Delay1 : UnitDelay  SampleTime=-1  HasFrameUpgradeWarning=on
  Voltage : Scope  NumInputPorts=2
  cell_model : MATLAB Function  TreatAsAtomicUnit=on
  V1 : Outport
  Z1 : Outport  Port=2
  irc1 : Outport  Port=3
  wires:
  Constant/1 -> cell_model/3(iR0)
  Unit Delay1/1 -> cell_model/5(irkp)
  cell_model/2(irkc) -> States/2, Unit Delay1/1, irc1/1
  Unit Delay/1 -> cell_model/4(zkp)
  Constant2/1 -> cell_model/1(T)
  Constant1/1 -> cell_model/2(deltaT)
  cell_model/1(vk) -> Voltage/1, V1/1
  cell_model/3(zkc) -> States/1, Unit Delay/1, Z1/1
  ik1/1 -> cell_model/6(ik)
  cell_model/4(OCV) -> Voltage/2

== system sim_battery_pack_simulink_18_11/SCM6/cell6 ==
  ik1 : Inport
  Constant : Constant  Value=R0
  Constant1 : Constant  Value=dt
  Constant2 : Constant  Value=T
  States : Scope  NumInputPorts=2
  Unit Delay : UnitDelay  InitialCondition=Z0(6,6)  SampleTime=-1  HasFrameUpgradeWarning=on
  Unit Delay1 : UnitDelay  SampleTime=-1  HasFrameUpgradeWarning=on
  Voltage : Scope  NumInputPorts=2
  cell_model : MATLAB Function  TreatAsAtomicUnit=on
  V1 : Outport
  Z1 : Outport  Port=2
  irc1 : Outport  Port=3
  wires:
  Constant/1 -> cell_model/3(iR0)
  Unit Delay1/1 -> cell_model/5(irkp)
  cell_model/2(irkc) -> States/2, Unit Delay1/1, irc1/1
  Unit Delay/1 -> cell_model/4(zkp)
  Constant2/1 -> cell_model/1(T)
  Constant1/1 -> cell_model/2(deltaT)
  cell_model/1(vk) -> Voltage/1, V1/1
  cell_model/3(zkc) -> States/1, Unit Delay/1, Z1/1
  ik1/1 -> cell_model/6(ik)
  cell_model/4(OCV) -> Voltage/2

== system sim_battery_pack_simulink_18_11/SCM6/cell7 ==
  ik1 : Inport
  Constant : Constant  Value=R0
  Constant1 : Constant  Value=dt
  Constant2 : Constant  Value=T
  States : Scope  NumInputPorts=2
  Unit Delay : UnitDelay  InitialCondition=Z0(7,6)  SampleTime=-1  HasFrameUpgradeWarning=on
  Unit Delay1 : UnitDelay  SampleTime=-1  HasFrameUpgradeWarning=on
  Voltage : Scope  NumInputPorts=2
  cell_model : MATLAB Function  TreatAsAtomicUnit=on
  V1 : Outport
  Z1 : Outport  Port=2
  irc1 : Outport  Port=3
  wires:
  cell_model/4(OCV) -> Voltage/2
  ik1/1 -> cell_model/6(ik)
  cell_model/3(zkc) -> Z1/1, Unit Delay/1, States/1
  cell_model/1(vk) -> V1/1, Voltage/1
  Constant1/1 -> cell_model/2(deltaT)
  Constant2/1 -> cell_model/1(T)
  Unit Delay/1 -> cell_model/4(zkp)
  cell_model/2(irkc) -> irc1/1, Unit Delay1/1, States/2
  Unit Delay1/1 -> cell_model/5(irkp)
  Constant/1 -> cell_model/3(iR0)

== system sim_battery_pack_simulink_18_11/SCM6/cell8 ==
  ik1 : Inport
  Constant : Constant  Value=R0
  Constant1 : Constant  Value=dt
  Constant2 : Constant  Value=T
  States : Scope  NumInputPorts=2
  Unit Delay : UnitDelay  InitialCondition=Z0(8,6)  SampleTime=-1  HasFrameUpgradeWarning=on
  Unit Delay1 : UnitDelay  SampleTime=-1  HasFrameUpgradeWarning=on
  Voltage : Scope  NumInputPorts=2
  cell_model : MATLAB Function  TreatAsAtomicUnit=on
  V1 : Outport
  Z1 : Outport  Port=2
  irc1 : Outport  Port=3
  wires:
  Constant/1 -> cell_model/3(iR0)
  Unit Delay1/1 -> cell_model/5(irkp)
  cell_model/2(irkc) -> States/2, Unit Delay1/1, irc1/1
  Unit Delay/1 -> cell_model/4(zkp)
  Constant2/1 -> cell_model/1(T)
  Constant1/1 -> cell_model/2(deltaT)
  cell_model/1(vk) -> Voltage/1, V1/1
  cell_model/3(zkc) -> States/1, Unit Delay/1, Z1/1
  ik1/1 -> cell_model/6(ik)
  cell_model/4(OCV) -> Voltage/2

== system sim_battery_pack_simulink_18_11/SCM6/cell9 ==
  ik1 : Inport
  Constant : Constant  Value=R0
  Constant1 : Constant  Value=dt
  Constant2 : Constant  Value=T
  States : Scope  NumInputPorts=2
  Unit Delay : UnitDelay  InitialCondition=Z0(9,6)  SampleTime=-1  HasFrameUpgradeWarning=on
  Unit Delay1 : UnitDelay  SampleTime=-1  HasFrameUpgradeWarning=on
  Voltage : Scope  NumInputPorts=2
  cell_model : MATLAB Function  TreatAsAtomicUnit=on
  V1 : Outport
  Z1 : Outport  Port=2
  irc1 : Outport  Port=3
  wires:
  cell_model/4(OCV) -> Voltage/2
  ik1/1 -> cell_model/6(ik)
  cell_model/3(zkc) -> Z1/1, Unit Delay/1, States/1
  cell_model/1(vk) -> V1/1, Voltage/1
  Constant1/1 -> cell_model/2(deltaT)
  Constant2/1 -> cell_model/1(T)
  Unit Delay/1 -> cell_model/4(zkp)
  cell_model/2(irkc) -> irc1/1, Unit Delay1/1, States/2
  Unit Delay1/1 -> cell_model/5(irkp)
  Constant/1 -> cell_model/3(iR0)

== system sim_battery_pack_simulink_18_11/SCM7/cell1 ==
  ik1 : Inport
  Constant : Constant  Value=R0
  Constant1 : Constant  Value=dt
  Constant2 : Constant  Value=T
  States : Scope  NumInputPorts=2
  Unit Delay : UnitDelay  InitialCondition=Z0(1,7)  SampleTime=-1  HasFrameUpgradeWarning=on
  Unit Delay1 : UnitDelay  SampleTime=-1  HasFrameUpgradeWarning=on
  Voltage : Scope  NumInputPorts=2
  cell_model : MATLAB Function  TreatAsAtomicUnit=on
  V1 : Outport
  Z1 : Outport  Port=2
  irc1 : Outport  Port=3
  wires:
  cell_model/4(OCV) -> Voltage/2
  ik1/1 -> cell_model/6(ik)
  cell_model/3(zkc) -> Z1/1, Unit Delay/1, States/1
  cell_model/1(vk) -> V1/1, Voltage/1
  Constant1/1 -> cell_model/2(deltaT)
  Constant2/1 -> cell_model/1(T)
  Unit Delay/1 -> cell_model/4(zkp)
  cell_model/2(irkc) -> irc1/1, Unit Delay1/1, States/2
  Unit Delay1/1 -> cell_model/5(irkp)
  Constant/1 -> cell_model/3(iR0)

== system sim_battery_pack_simulink_18_11/SCM7/cell10 ==
  ik1 : Inport
  Constant : Constant  Value=R0
  Constant1 : Constant  Value=dt
  Constant2 : Constant  Value=T
  States : Scope  NumInputPorts=2
  Unit Delay : UnitDelay  InitialCondition=Z0(10,7)  SampleTime=-1  HasFrameUpgradeWarning=on
  Unit Delay1 : UnitDelay  SampleTime=-1  HasFrameUpgradeWarning=on
  Voltage : Scope  NumInputPorts=2
  cell_model : MATLAB Function  TreatAsAtomicUnit=on
  V1 : Outport
  Z1 : Outport  Port=2
  irc1 : Outport  Port=3
  wires:
  cell_model/4(OCV) -> Voltage/2
  ik1/1 -> cell_model/6(ik)
  cell_model/3(zkc) -> Z1/1, Unit Delay/1, States/1
  cell_model/1(vk) -> V1/1, Voltage/1
  Constant1/1 -> cell_model/2(deltaT)
  Constant2/1 -> cell_model/1(T)
  Unit Delay/1 -> cell_model/4(zkp)
  cell_model/2(irkc) -> irc1/1, Unit Delay1/1, States/2
  Unit Delay1/1 -> cell_model/5(irkp)
  Constant/1 -> cell_model/3(iR0)

== system sim_battery_pack_simulink_18_11/SCM7/cell11 ==
  ik1 : Inport
  Constant : Constant  Value=R0
  Constant1 : Constant  Value=dt
  Constant2 : Constant  Value=T
  States : Scope  NumInputPorts=2
  Unit Delay : UnitDelay  InitialCondition=Z0(11,7)  SampleTime=-1  HasFrameUpgradeWarning=on
  Unit Delay1 : UnitDelay  SampleTime=-1  HasFrameUpgradeWarning=on
  Voltage : Scope  NumInputPorts=2
  cell_model : MATLAB Function  TreatAsAtomicUnit=on
  V1 : Outport
  Z1 : Outport  Port=2
  irc1 : Outport  Port=3
  wires:
  Constant/1 -> cell_model/3(iR0)
  Unit Delay1/1 -> cell_model/5(irkp)
  cell_model/2(irkc) -> States/2, Unit Delay1/1, irc1/1
  Unit Delay/1 -> cell_model/4(zkp)
  Constant2/1 -> cell_model/1(T)
  Constant1/1 -> cell_model/2(deltaT)
  cell_model/1(vk) -> Voltage/1, V1/1
  cell_model/3(zkc) -> States/1, Unit Delay/1, Z1/1
  ik1/1 -> cell_model/6(ik)
  cell_model/4(OCV) -> Voltage/2

== system sim_battery_pack_simulink_18_11/SCM7/cell12 ==
  ik1 : Inport
  Constant : Constant  Value=R0
  Constant1 : Constant  Value=dt
  Constant2 : Constant  Value=T
  States : Scope  NumInputPorts=2
  Unit Delay : UnitDelay  InitialCondition=Z0(12,7)  SampleTime=-1  HasFrameUpgradeWarning=on
  Unit Delay1 : UnitDelay  SampleTime=-1  HasFrameUpgradeWarning=on
  Voltage : Scope  NumInputPorts=2
  cell_model : MATLAB Function  TreatAsAtomicUnit=on
  V1 : Outport
  Z1 : Outport  Port=2
  irc1 : Outport  Port=3
  wires:
  Constant/1 -> cell_model/3(iR0)
  Unit Delay1/1 -> cell_model/5(irkp)
  cell_model/2(irkc) -> States/2, Unit Delay1/1, irc1/1
  Unit Delay/1 -> cell_model/4(zkp)
  Constant2/1 -> cell_model/1(T)
  Constant1/1 -> cell_model/2(deltaT)
  cell_model/1(vk) -> Voltage/1, V1/1
  cell_model/3(zkc) -> States/1, Unit Delay/1, Z1/1
  ik1/1 -> cell_model/6(ik)
  cell_model/4(OCV) -> Voltage/2

== system sim_battery_pack_simulink_18_11/SCM7/cell2 ==
  ik1 : Inport
  Constant : Constant  Value=R0
  Constant1 : Constant  Value=dt
  Constant2 : Constant  Value=T
  States : Scope  NumInputPorts=2
  Unit Delay : UnitDelay  InitialCondition=Z0(2,7)  SampleTime=-1  HasFrameUpgradeWarning=on
  Unit Delay1 : UnitDelay  SampleTime=-1  HasFrameUpgradeWarning=on
  Voltage : Scope  NumInputPorts=2
  cell_model : MATLAB Function  TreatAsAtomicUnit=on
  V1 : Outport
  Z1 : Outport  Port=2
  irc1 : Outport  Port=3
  wires:
  cell_model/4(OCV) -> Voltage/2
  ik1/1 -> cell_model/6(ik)
  cell_model/3(zkc) -> Z1/1, Unit Delay/1, States/1
  cell_model/1(vk) -> V1/1, Voltage/1
  Constant1/1 -> cell_model/2(deltaT)
  Constant2/1 -> cell_model/1(T)
  Unit Delay/1 -> cell_model/4(zkp)
  cell_model/2(irkc) -> irc1/1, Unit Delay1/1, States/2
  Unit Delay1/1 -> cell_model/5(irkp)
  Constant/1 -> cell_model/3(iR0)

== system sim_battery_pack_simulink_18_11/SCM7/cell3 ==
  ik1 : Inport
  Constant : Constant  Value=R0
  Constant1 : Constant  Value=dt
  Constant2 : Constant  Value=T
  States : Scope  NumInputPorts=2
  Unit Delay : UnitDelay  InitialCondition=Z0(3,7)  SampleTime=-1  HasFrameUpgradeWarning=on
  Unit Delay1 : UnitDelay  SampleTime=-1  HasFrameUpgradeWarning=on
  Voltage : Scope  NumInputPorts=2
  cell_model : MATLAB Function  TreatAsAtomicUnit=on
  V1 : Outport
  Z1 : Outport  Port=2
  irc1 : Outport  Port=3
  wires:
  Constant/1 -> cell_model/3(iR0)
  Unit Delay1/1 -> cell_model/5(irkp)
  cell_model/2(irkc) -> States/2, Unit Delay1/1, irc1/1
  Unit Delay/1 -> cell_model/4(zkp)
  Constant2/1 -> cell_model/1(T)
  Constant1/1 -> cell_model/2(deltaT)
  cell_model/1(vk) -> Voltage/1, V1/1
  cell_model/3(zkc) -> States/1, Unit Delay/1, Z1/1
  ik1/1 -> cell_model/6(ik)
  cell_model/4(OCV) -> Voltage/2

== system sim_battery_pack_simulink_18_11/SCM7/cell4 ==
  ik1 : Inport
  Constant : Constant  Value=R0
  Constant1 : Constant  Value=dt
  Constant2 : Constant  Value=T
  States : Scope  NumInputPorts=2
  Unit Delay : UnitDelay  InitialCondition=Z0(4,7)  SampleTime=-1  HasFrameUpgradeWarning=on
  Unit Delay1 : UnitDelay  SampleTime=-1  HasFrameUpgradeWarning=on
  Voltage : Scope  NumInputPorts=2
  cell_model : MATLAB Function  TreatAsAtomicUnit=on
  V1 : Outport
  Z1 : Outport  Port=2
  irc1 : Outport  Port=3
  wires:
  Constant/1 -> cell_model/3(iR0)
  Unit Delay1/1 -> cell_model/5(irkp)
  cell_model/2(irkc) -> States/2, Unit Delay1/1, irc1/1
  Unit Delay/1 -> cell_model/4(zkp)
  Constant2/1 -> cell_model/1(T)
  Constant1/1 -> cell_model/2(deltaT)
  cell_model/1(vk) -> Voltage/1, V1/1
  cell_model/3(zkc) -> States/1, Unit Delay/1, Z1/1
  ik1/1 -> cell_model/6(ik)
  cell_model/4(OCV) -> Voltage/2

== system sim_battery_pack_simulink_18_11/SCM7/cell5 ==
  ik1 : Inport
  Constant : Constant  Value=R0
  Constant1 : Constant  Value=dt
  Constant2 : Constant  Value=T
  States : Scope  NumInputPorts=2
  Unit Delay : UnitDelay  InitialCondition=Z0(5,7)  SampleTime=-1  HasFrameUpgradeWarning=on
  Unit Delay1 : UnitDelay  SampleTime=-1  HasFrameUpgradeWarning=on
  Voltage : Scope  NumInputPorts=2
  cell_model : MATLAB Function  TreatAsAtomicUnit=on
  V1 : Outport
  Z1 : Outport  Port=2
  irc1 : Outport  Port=3
  wires:
  cell_model/4(OCV) -> Voltage/2
  ik1/1 -> cell_model/6(ik)
  cell_model/3(zkc) -> Z1/1, Unit Delay/1, States/1
  cell_model/1(vk) -> V1/1, Voltage/1
  Constant1/1 -> cell_model/2(deltaT)
  Constant2/1 -> cell_model/1(T)
  Unit Delay/1 -> cell_model/4(zkp)
  cell_model/2(irkc) -> irc1/1, Unit Delay1/1, States/2
  Unit Delay1/1 -> cell_model/5(irkp)
  Constant/1 -> cell_model/3(iR0)
